simulink model "vbyf"  (R2024b)
settings: Solver=VariableStepAuto  StartTime=0.0  StopTime=10.0  RelTol=1e-3
values from neighbouring files (symbols this model uses):
  pmsm =     [foc.mat]    (also in inverter.mat; speed_control.mat; vbyf.mat)
  Ts = 2.5e-05    [foc.mat]    (also in inverter.mat; speed_control.mat; vbyf.mat)
libraries: mcbplantlib x1, autolibpmsminterior x1, mcbpmsmvflib x1
settings Model: Creator=realf  LastModifiedBy=realf

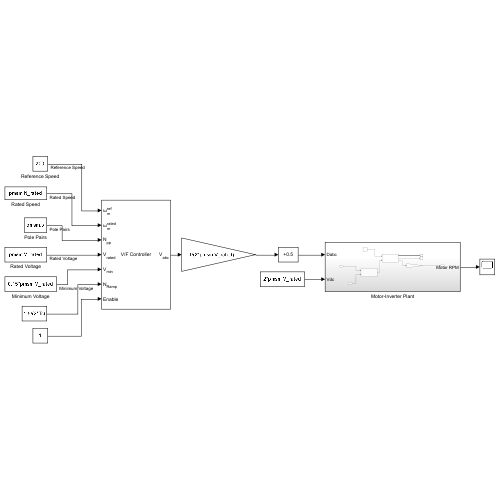
[thumbnail: Simulink's stored preview of the top-level diagram]
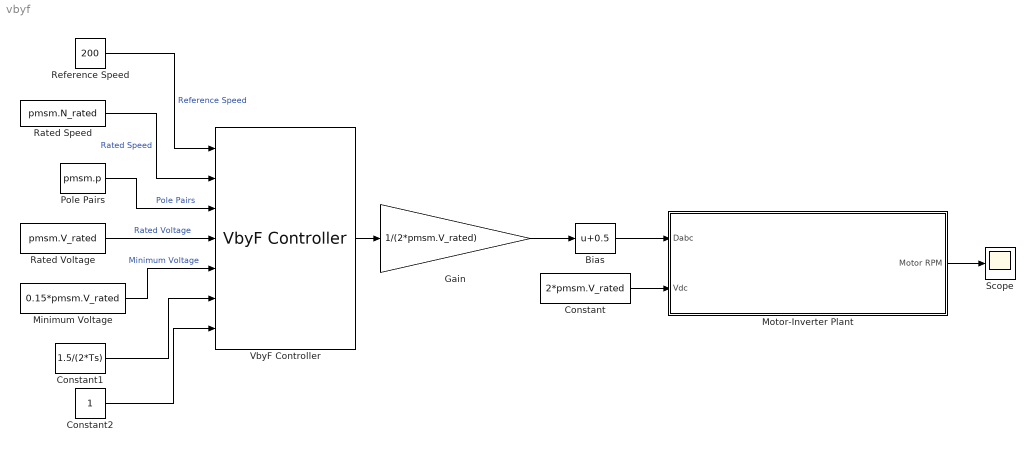
== system vbyf ==
  Bias : Bias  Bias=0.5  SaturateOnIntegerOverflow=off
  Constant : Constant  Value=2*pmsm.V_rated
  Constant1 : Constant  Value=1.5/(2*Ts)
  Constant2 : Constant
  Gain : Gain  Gain=1/(2*pmsm.V_rated)
  Minimum Voltage : Constant  Value=0.15*pmsm.V_rated
  Motor-Inverter Plant : Subsystem
  Pole Pairs : Constant  Value=pmsm.p
  Rated Speed : Constant  Value=pmsm.N_rated
  Rated Voltage : Constant  Value=pmsm.V_rated
  Reference Speed : Constant  Value=200
  Scope : Scope
  VbyF Controller : mcbpmsmvflib/VbyF Controller  SpeedUnit=RPM  BaseSpeed=1200  Ts=2*Ts
      settings: LibrarySourceBlock=mcblib/Controls/Controllers/VbyF Controller
  wires:
  Constant2/1 -> VbyF Controller/7
  Rated Speed/1 -> VbyF Controller/2  "Rated Speed"
  Reference Speed/1 -> VbyF Controller/1  "Reference Speed"
  Rated Voltage/1 -> VbyF Controller/4  "Rated Voltage"
  Pole Pairs/1 -> VbyF Controller/3  "Pole Pairs"
  Minimum Voltage/1 -> VbyF Controller/5  "Minimum Voltage"
  Constant1/1 -> VbyF Controller/6
  VbyF Controller/1 -> Gain/1
  Gain/1 -> Bias/1
  Bias/1 -> Motor-Inverter Plant/1(Dabc)
  Constant/1 -> Motor-Inverter Plant/2(Vdc)
  Motor-Inverter Plant/1(Motor RPM) -> Scope/1

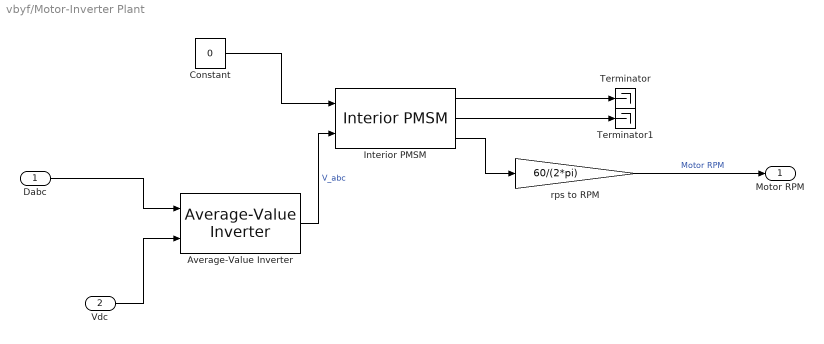
== system vbyf/Motor-Inverter Plant ==
  Dabc : Inport
  Vdc : Inport  Port=2
  Average-Value Inverter : mcbplantlib/Average-Value Inverter
  Constant : Constant  Value=0
  Interior PMSM : autolibpmsminterior/Interior PMSM  port_config=Torque  sim_type=Discrete  Ts=Ts  P=pmsm.p  Rs=pmsm.Rs  Ldq=[pmsm.Ld, pmsm.Lq]  KConstText=Permanent flux linkage constant (lambda_pm):  lambda_pm=pmsm.FluxPM  Ke=159.9771  mechanical=[pmsm.J, 0, 0]  idq0=[0 0]  theta_init=0  omega_init=0  KConst=pmsm.FluxPM  lambda_pm_calc=pmsm.FluxPM  Kt=0.07  RefBlkName='autolibpmsminterior/Interior PMSM'  aMode=5
  Terminator : Terminator
  Terminator1 : Terminator
  rps to RPM : Gain  Gain=60/(2*pi)
  Motor RPM : Outport
  wires:
  rps to RPM/1 -> Motor RPM/1  "Motor RPM"
  Interior PMSM/1 -> Terminator/1
  Interior PMSM/2 -> Terminator1/1
  Vdc/1 -> Average-Value Inverter/2
  Dabc/1 -> Average-Value Inverter/1
  Average-Value Inverter/1 -> Interior PMSM/2  "V_abc"
  Interior PMSM/3 -> rps to RPM/1
  Constant/1 -> Interior PMSM/1
